simulink model "IM_resistive_load"  (R2014a)
settings: Solver=ode45  StartTime=0.0  StopTime=4  RelTol=1e-3
libraries: powerlib x14, simulink_extras x9
settings Model: Creator=Divya M  LastModifiedBy=Divya M

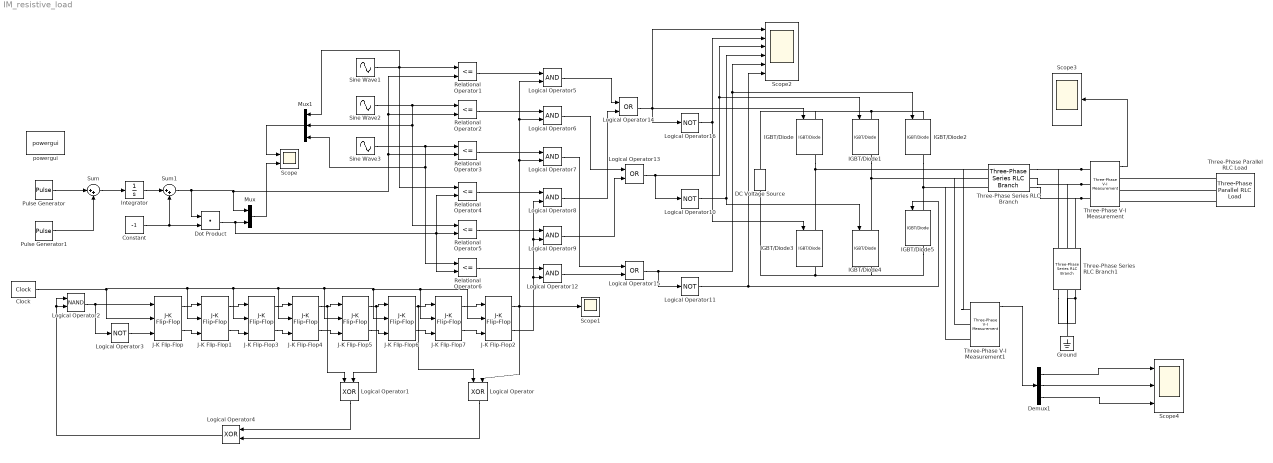
== system IM_resistive_load ==
  Clock : simulink_extras/Flip Flops/Clock  period=1/(3e3)
  Constant : Constant  Value=-1
  DC Voltage Source : powerlib/Electrical Sources/DC Voltage Source  Amplitude=400  Measurements=None
  Demux1 : Demux  Outputs=3
  Dot Product : DotProduct  InputSameDT=on  OutDataTypeStr=Inherit: Inherit via internal rule
  Ground : powerlib/Elements/Ground  LConnTagsString=a
  IGBT/Diode{,1..5} (6 alike) : powerlib/Power Electronics/IGBT//Diode  Ron=1e-3  Rs=1e5  Cs=inf  Measurements=on
  Integrator : Integrator
  J-K Flip-Flop{,1..7} (8 alike) : simulink_extras/Flip Flops/J-K Flip-Flop  initial_condition=0
  Logical Operator : Logic  Operator=XOR  AllPortsSameDT=off  OutDataTypeStr=boolean
  Logical Operator1 : Logic  Operator=XOR  AllPortsSameDT=off  OutDataTypeStr=boolean
  Logical Operator{3,10..11,16} (4 alike) : Logic  Operator=NOT  AllPortsSameDT=off  OutDataTypeStr=boolean
  Logical Operator{5..9,12} (6 alike) : Logic  AllPortsSameDT=off  OutDataTypeStr=boolean
  Logical Operator13 : Logic  Operator=OR  AllPortsSameDT=off  OutDataTypeStr=boolean
  Logical Operator14 : Logic  Operator=OR  AllPortsSameDT=off  OutDataTypeStr=boolean
  Logical Operator15 : Logic  Operator=OR  AllPortsSameDT=off  OutDataTypeStr=boolean
  Logical Operator2 : Logic  Operator=NAND  AllPortsSameDT=off  OutDataTypeStr=boolean
  Logical Operator4 : Logic  Operator=XOR  AllPortsSameDT=off  OutDataTypeStr=boolean
  Mux : Mux  Inputs=2
  Mux1 : Mux  Inputs=3
  Pulse Generator : DiscretePulseGenerator  PulseType=Time based  Amplitude=12000  Period=1e-3/3  PulseWidth=50
  Pulse Generator1 : DiscretePulseGenerator  PulseType=Time based  Amplitude=-12000  Period=1/3e3  PulseWidth=50  PhaseDelay=1/6e3
  Relational Operator{1..6} (6 alike) : RelationalOperator  Operator=<=  OutDataTypeStr=boolean
  Scope : Scope  NumInputPorts=2
      settings: YMin=-1.2~-0.2  YMax=1.2~1.2
  Scope1 : Scope
      settings: YMin=-1.2  YMax=1.2  MaxDataPoints=5000000
  Scope2 : Scope  NumInputPorts=6
      settings: YMin=-0.2~-0.2~-0.2~-0.2~-0.2~-0.2  YMax=1.2~1.2~1.2~1.2~1.2~1.2  SaveName=ScopeData2
  Scope3 : Scope
      settings: YMin=-0.2  YMax=1.2  SaveName=ScopeData3  MaxDataPoints=500000
  Scope4 : Scope  NumInputPorts=3
      settings: YMin=-0.2~-0.2~-0.2  YMax=1.2~1.2~1.2  SaveName=ScopeData4  MaxDataPoints=500000
  Sine Wave1 : Sin  Frequency=314  SampleTime=0
  Sine Wave2 : Sin  Frequency=314  Phase=(2*pi)/3  SampleTime=0
  Sine Wave3 : Sin  Frequency=314  Phase=(4*pi)/3  SampleTime=0
  Sum : Sum  Inputs=|++
  Sum1 : Sum  Inputs=|++
  Three-Phase Parallel RLC Load : powerlib/Elements/Three-Phase Parallel RLC Load  LConnTagsString=A|B|C  Configuration=Y (grounded)  NominalVoltage=400*1.73  NominalFrequency=50  ActivePower=1e3  InductivePower=0  CapacitivePower=0  Measurements=None  LoadType=constant Z
  Three-Phase Series RLC Branch : powerlib/Elements/Three-Phase Series RLC Branch  LConnTagsString=A|B|C  RConnTagsString=A|B|C  BranchType=L  Resistance=1  Inductance=10  Capacitance=1e-6  Measurements=None
  Three-Phase Series RLC Branch1 : powerlib/Elements/Three-Phase Series RLC Branch  LConnTagsString=A|B|C  RConnTagsString=A|B|C  BranchType=C  Resistance=1  Inductance=10  Capacitance=1e-6  Measurements=None
  Three-Phase V-I Measurement : powerlib/Measurements/Three-Phase V-I Measurement  VoltageMeasurement=phase-to-phase  SetLabelV=off  LabelV=Vabc  Vpu=off  VpuLL=off  CurrentMeasurement=no  SetLabelI=off  LabelI=Iabc  Ipu=off  Pbase=100e6  Vbase=500e3  OutputType=Complex  PhasorSimulation=off  PSBequivalent=0
  Three-Phase V-I Measurement1 : powerlib/Measurements/Three-Phase V-I Measurement  VoltageMeasurement=phase-to-phase  SetLabelV=off  LabelV=Vabc  Vpu=off  VpuLL=off  CurrentMeasurement=no  SetLabelI=off  LabelI=Iabc  Ipu=off  Pbase=100e6  Vbase=500e3  OutputType=Complex  PhasorSimulation=off  PSBequivalent=0
  powergui : powerlib/powergui  Priority=1  SimulationMode=Continuous  SolverType=Tustin  SampleTime=50e-6  frequency=60  SPID=off  DisableSnubberDevices=off  DisableRonSwitches=off  DisableVfSwitches=off  SwTol=0  Interpol=off  DisplayEquations=off  Ts=0  methode=off  frequencyindice=0  Pbase=100e6  ErrMax=1e-4  Iterations=50  UnitsV=kV  UnitsW=MW  FunctionMessages=off  echomessages=off  HookPort=off  EnableUseOfTLC=off  x0status=blocks  RestoreLinks=warning  ResistiveCurrentMeasurement=off  Frange=[0:2:500]  Ylog=off  Xlog=on  ShowGrid=off  save=off  variable=ZData  structure=0  ZoomFFT=off  StartTime=0.0  cycles=1  DisplayStyle=1  fundamental=60  FreqAxis=off  MaxFrequency=1000  frequencyindicesteady=1  RmsSteady=1  display=off
  wires:
  Pulse Generator/1 -> Sum/1
  Pulse Generator1/1 -> Sum/2
  Sum/1 -> Integrator/1
  Integrator/1 -> Sum1/1
  Constant/1 -> Dot Product/2, Sum1/2
  Logical Operator2/1 -> Logical Operator3/1, J-K Flip-Flop/1
  Logical Operator3/1 -> J-K Flip-Flop/3
  J-K Flip-Flop/1 -> J-K Flip-Flop1/1
  J-K Flip-Flop/2 -> J-K Flip-Flop1/3
  J-K Flip-Flop1/1 -> J-K Flip-Flop3/1
  J-K Flip-Flop1/2 -> J-K Flip-Flop3/3
  J-K Flip-Flop3/1 -> J-K Flip-Flop4/1
  J-K Flip-Flop3/2 -> J-K Flip-Flop4/3
  J-K Flip-Flop4/1 -> J-K Flip-Flop5/1, Logical Operator1/1
  J-K Flip-Flop4/2 -> J-K Flip-Flop5/3
  J-K Flip-Flop5/1 -> J-K Flip-Flop6/1, Logical Operator1/2
  J-K Flip-Flop5/2 -> J-K Flip-Flop6/3
  J-K Flip-Flop6/1 -> Logical Operator/1, J-K Flip-Flop7/1
  J-K Flip-Flop6/2 -> J-K Flip-Flop7/3
  J-K Flip-Flop7/1 -> J-K Flip-Flop2/1
  J-K Flip-Flop7/2 -> J-K Flip-Flop2/3
  Clock/1 -> J-K Flip-Flop3/2, J-K Flip-Flop2/2, J-K Flip-Flop7/2, J-K Flip-Flop6/2, J-K Flip-Flop5/2, J-K Flip-Flop4/2, J-K Flip-Flop1/2, J-K Flip-Flop/2
  Logical Operator1/1 -> Logical Operator4/1
  Logical Operator/1 -> Logical Operator4/2
  Logical Operator4/1 -> Logical Operator2/2, Logical Operator2/1
  Sine Wave1/1 -> Mux1/1, Relational Operator1/1, Relational Operator4/1
  Sine Wave2/1 -> Relational Operator2/1, Mux1/2, Relational Operator5/1
  Sine Wave3/1 -> Relational Operator3/1, Relational Operator6/1, Mux1/3
  Sum1/1 -> Relational Operator3/2, Relational Operator2/2, Relational Operator1/2, Mux/1, Dot Product/1
  Dot Product/1 -> Relational Operator5/2, Relational Operator6/2, Relational Operator4/2, Mux/2
  Relational Operator1/1 -> Logical Operator5/1
  Relational Operator2/1 -> Logical Operator6/1
  Relational Operator3/1 -> Logical Operator7/1
  Relational Operator4/1 -> Logical Operator8/1
  Relational Operator5/1 -> Logical Operator9/1
  Relational Operator6/1 -> Logical Operator12/1
  J-K Flip-Flop2/1 -> Logical Operator/2, Logical Operator7/2, Logical Operator6/2, Logical Operator5/2, Scope1/1
  J-K Flip-Flop2/2 -> Logical Operator12/2, Logical Operator8/2, Logical Operator9/2
  Logical Operator5/1 -> Logical Operator14/1
  Logical Operator8/1 -> Logical Operator14/2
  Logical Operator6/1 -> Logical Operator13/1
  Logical Operator9/1 -> Logical Operator13/2
  Logical Operator7/1 -> Logical Operator15/1
  Logical Operator12/1 -> Logical Operator15/2
  Logical Operator14/1 -> Scope2/1, IGBT/Diode/1, Logical Operator16/1
  Logical Operator15/1 -> IGBT/Diode2/1, Scope2/5, Logical Operator11/1
  Logical Operator13/1 -> Logical Operator10/1, IGBT/Diode1/1, Scope2/3
  Logical Operator16/1 -> IGBT/Diode3/1, Scope2/2
  Logical Operator10/1 -> IGBT/Diode4/1, Scope2/4
  Logical Operator11/1 -> IGBT/Diode5/1, Scope2/6
  Mux/1 -> Scope/2
  Mux1/1 -> Scope/1
  Three-Phase V-I Measurement/1 -> Scope3/1
  Three-Phase V-I Measurement1/1 -> Demux1/1
  Demux1/2 -> Scope4/2
  Demux1/1 -> Scope4/1
  Demux1/3 -> Scope4/3
  connections:
  IGBT/Diode1/LConn1 -- IGBT/Diode2/LConn1 -- DC Voltage Source/RConn1 -- IGBT/Diode/LConn1
  IGBT/Diode3/RConn1 -- DC Voltage Source/LConn1 -- IGBT/Diode5/RConn1 -- IGBT/Diode4/RConn1
  IGBT/Diode2/RConn1 -- Three-Phase V-I Measurement1/LConn3 -- Three-Phase Series RLC Branch/LConn3 -- IGBT/Diode5/LConn1
  IGBT/Diode1/RConn1 -- Three-Phase V-I Measurement1/LConn2 -- Three-Phase Series RLC Branch/LConn2 -- IGBT/Diode4/LConn1
  IGBT/Diode/RConn1 -- Three-Phase Series RLC Branch/LConn1 -- Three-Phase V-I Measurement1/LConn1 -- IGBT/Diode3/LConn1
  Three-Phase V-I Measurement/LConn1 -- Three-Phase Series RLC Branch/RConn1 -- Three-Phase Series RLC Branch1/LConn1
  Three-Phase V-I Measurement/LConn2 -- Three-Phase Series RLC Branch/RConn2 -- Three-Phase Series RLC Branch1/LConn2
  Three-Phase V-I Measurement/LConn3 -- Three-Phase Series RLC Branch/RConn3 -- Three-Phase Series RLC Branch1/LConn3
  Three-Phase Series RLC Branch1/RConn3 -- Three-Phase Series RLC Branch1/RConn1 -- Ground/LConn1 -- Three-Phase Series RLC Branch1/RConn2
  Three-Phase Parallel RLC Load/LConn3 -- Three-Phase V-I Measurement/RConn3
  Three-Phase Parallel RLC Load/LConn2 -- Three-Phase V-I Measurement/RConn2
  Three-Phase Parallel RLC Load/LConn1 -- Three-Phase V-I Measurement/RConn1
